simulink model "SHM_900HZ_TG190428test"  (Simulink 7.7)
settings: Solver=ode113  SolverMode=SingleTasking  StartTime=0.0  StopTime=3  RelTol=0.5e-4
undefined symbols (not defined in the file): D11, Delta, SHM900
libraries: powerlib x37, powerlib_extras x22, simulink x6, simulink_extras x1
(part 2 of 2)

== system SHM_900HZ_TG190428test/Controller/PLL/P-I ==
  X : Inport
  Data Type Conversion : DataTypeConversion  SampleTime=TA
  Data Type Conversion3 : DataTypeConversion  SampleTime=TA
  INT1 : Subsystem
  K_i : Gain  Gain=10  SampleTime=TA
  K_p : Gain  SampleTime=TA
  Ki2 : Constant  Value=0.2
  Ki4 : Constant  Value=-0.2
  Logical Operator : Logic  Operator=NOR  AllPortsSameDT=off  OutDataTypeStr=boolean  SampleTime=TA
  Relational Operator : RelationalOperator  OutDataTypeStr=boolean  ZeroCross=off  SampleTime=TA
  Relational Operator1 : RelationalOperator  Operator=<=  OutDataTypeStr=boolean  ZeroCross=off  SampleTime=TA
  Sum2 : Sum  SampleTime=TA
  Switch3 : Switch  Threshold=0.5  ZeroCross=off  SampleTime=TA
  Switch4 : Switch  Threshold=0.5  ZeroCross=off  SampleTime=TA
  Unit Delay : UnitDelay  SampleTime=TA
  Y : Outport
  wires:
  K_p/1 -> Sum2/1
  Sum2/1 -> Relational Operator/1, Switch3/3
  K_i/1 -> INT1/1(x)
  INT1/1(y) -> Sum2/2
  Data Type Conversion/1 -> Switch3/2
  Ki2/1 -> Switch3/1, Relational Operator/2
  Relational Operator/1 -> Data Type Conversion/1, Logical Operator/2
  Switch3/1 -> Switch4/3, Relational Operator1/1
  Ki4/1 -> Switch4/1, Relational Operator1/2
  Relational Operator1/1 -> Data Type Conversion3/1, Logical Operator/1
  Data Type Conversion3/1 -> Switch4/2
  Logical Operator/1 -> Unit Delay/1
  Unit Delay/1 -> INT1/2(S)
  X/1 -> K_p/1, K_i/1
  Switch4/1 -> Y/1

== system SHM_900HZ_TG190428test/Controller/Regulator1/1st order delay1 ==
  x : Inport
  Kd_1 : Gain  Gain=TA/0.005  SampleTime=TA
  Kd_2 : Gain  Gain=0.5  SampleTime=TA
  Sum1 : Sum  SampleTime=TA
  Sum4 : Sum  Inputs=+-  SampleTime=TA
  Sum6 : Sum  SampleTime=TA
  Unit Delay1 : UnitDelay  SampleTime=TA
  y : Outport
  wires:
  Sum4/1 -> Kd_1/1
  Kd_1/1 -> Sum6/1
  Sum6/1 -> Unit Delay1/1, Sum1/1
  Unit Delay1/1 -> Sum6/2, Sum4/2, Sum1/2
  x/1 -> Sum4/1
  Sum1/1 -> Kd_2/1
  Kd_2/1 -> y/1

== system SHM_900HZ_TG190428test/Controller/Regulator1/1st order delay2 ==
  x : Inport
  Kd_1 : Gain  Gain=TA/0.05  SampleTime=TA
  Kd_2 : Gain  Gain=0.5  SampleTime=TA
  Sum1 : Sum  SampleTime=TA
  Sum4 : Sum  Inputs=+-  SampleTime=TA
  Sum6 : Sum  SampleTime=TA
  Unit Delay1 : UnitDelay  SampleTime=TA
  y : Outport
  wires:
  Sum4/1 -> Kd_1/1
  Kd_1/1 -> Sum6/1
  Sum6/1 -> Unit Delay1/1, Sum1/1
  Unit Delay1/1 -> Sum6/2, Sum4/2, Sum1/2
  x/1 -> Sum4/1
  Sum1/1 -> Kd_2/1
  Kd_2/1 -> y/1

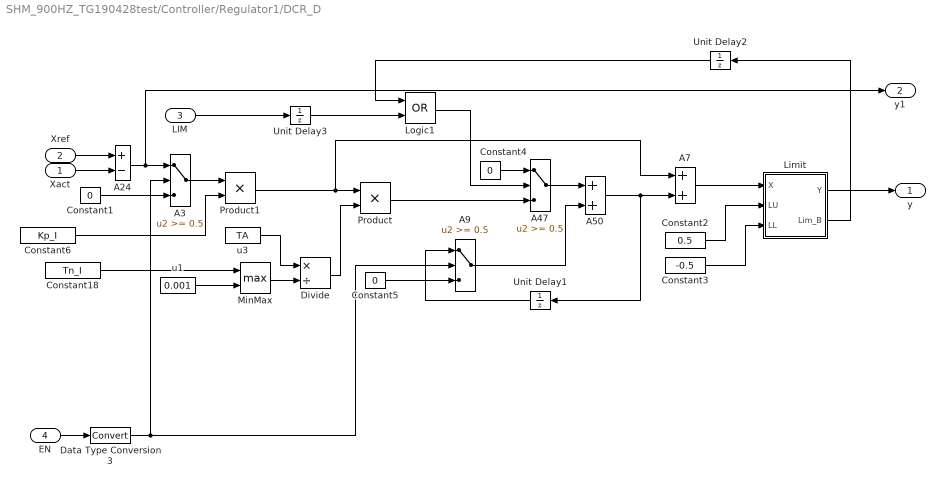
== system SHM_900HZ_TG190428test/Controller/Regulator1/DCR_D ==
  Xact : Inport
  Xref : Inport  Port=2
  LIM : Inport  Port=3
  EN : Inport  Port=4
  A24 : Sum  Inputs=+-  SampleTime=TA
  A3 : Switch  Threshold=0.5  ZeroCross=off
  A47 : Switch  Threshold=0.5  ZeroCross=off
  A50 : Sum  SampleTime=TA
  A7 : Sum  InputSameDT=on
  A9 : Switch  Threshold=0.5  ZeroCross=off
  Constant1 : Constant  Value=0
  Constant18 : Constant  Value=Tn_I
  Constant2 : Constant  Value=0.5
  Constant3 : Constant  Value=-0.5
  Constant4 : Constant  Value=0
  Constant5 : Constant  Value=0
  Constant6 : Constant  Value=Kp_I
  Data Type Conversion3 : DataTypeConversion
  Divide : Product  Inputs=*/
  Limit : Subsystem
  Logic1 : Logic  Operator=OR  AllPortsSameDT=off  OutDataTypeStr=boolean
  MinMax : MinMax  Function=max  Inputs=2
  Product : Product  RndMeth=Zero
  Product1 : Product  RndMeth=Zero
  Unit Delay1 : UnitDelay  SampleTime=-1
  Unit Delay2 : UnitDelay  SampleTime=-1
  Unit Delay3 : UnitDelay  SampleTime=-1
  u1 : Constant  Value=0.001  SampleTime=-1
  u3 : Constant  Value=TA  SampleTime=-1
  y : Outport
  y1 : Outport  Port=2
  wires:
  Divide/1 -> Product/2
  MinMax/1 -> Divide/2
  u1/1 -> MinMax/2
  u3/1 -> Divide/1
  Constant18/1 -> MinMax/1
  Data Type Conversion3/1 -> A3/2, A9/2
  Xact/1 -> A24/2
  Xref/1 -> A24/1
  A24/1 -> A3/1, y1/1
  Constant1/1 -> A3/3
  A3/1 -> Product1/1
  Constant6/1 -> Product1/2
  Product1/1 -> A7/1, Product/1
  Product/1 -> A47/3
  Limit/1(Y) -> y/1
  EN/1 -> Data Type Conversion3/1
  Unit Delay1/1 -> A9/1
  Constant5/1 -> A9/3
  Constant4/1 -> A47/1
  A47/1 -> A50/1
  A9/1 -> A50/2
  A50/1 -> A7/2, Unit Delay1/1
  A7/1 -> Limit/1(X)
  Constant2/1 -> Limit/2(LU)
  Constant3/1 -> Limit/3(LL)
  Limit/2(Lim_B) -> Unit Delay2/1
  Logic1/1 -> A47/2
  Unit Delay2/1 -> Logic1/1
  Unit Delay3/1 -> Logic1/2
  LIM/1 -> Unit Delay3/1

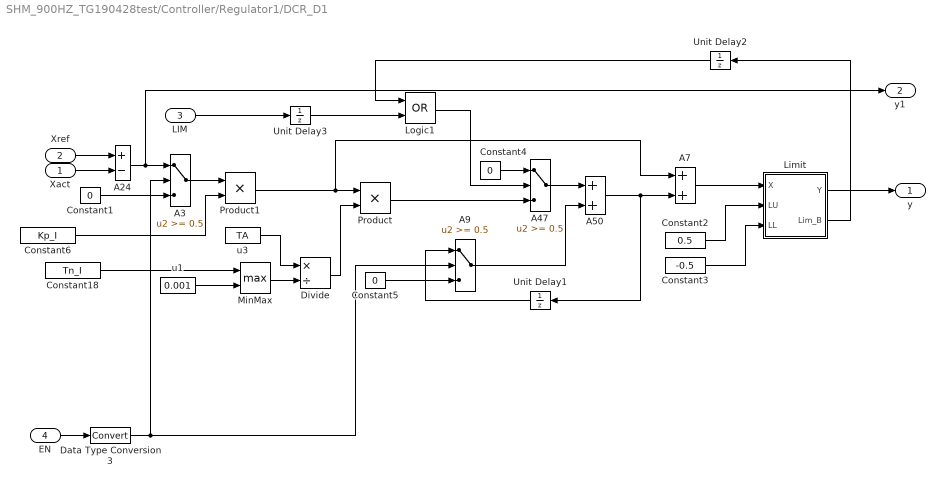
== system SHM_900HZ_TG190428test/Controller/Regulator1/DCR_D1 ==
  Xact : Inport
  Xref : Inport  Port=2
  LIM : Inport  Port=3
  EN : Inport  Port=4
  A24 : Sum  Inputs=+-  SampleTime=TA
  A3 : Switch  Threshold=0.5  ZeroCross=off
  A47 : Switch  Threshold=0.5  ZeroCross=off
  A50 : Sum  SampleTime=TA
  A7 : Sum  InputSameDT=on
  A9 : Switch  Threshold=0.5  ZeroCross=off
  Constant1 : Constant  Value=0
  Constant18 : Constant  Value=Tn_I
  Constant2 : Constant  Value=0.5
  Constant3 : Constant  Value=-0.5
  Constant4 : Constant  Value=0
  Constant5 : Constant  Value=0
  Constant6 : Constant  Value=Kp_I
  Data Type Conversion3 : DataTypeConversion
  Divide : Product  Inputs=*/
  Limit : Subsystem
  Logic1 : Logic  Operator=OR  AllPortsSameDT=off  OutDataTypeStr=boolean
  MinMax : MinMax  Function=max  Inputs=2
  Product : Product  RndMeth=Zero
  Product1 : Product  RndMeth=Zero
  Unit Delay1 : UnitDelay  SampleTime=-1
  Unit Delay2 : UnitDelay  SampleTime=-1
  Unit Delay3 : UnitDelay  SampleTime=-1
  u1 : Constant  Value=0.001  SampleTime=-1
  u3 : Constant  Value=TA  SampleTime=-1
  y : Outport
  y1 : Outport  Port=2
  wires:
  LIM/1 -> Unit Delay3/1
  Unit Delay3/1 -> Logic1/2
  Unit Delay2/1 -> Logic1/1
  Logic1/1 -> A47/2
  Limit/2(Lim_B) -> Unit Delay2/1
  Constant3/1 -> Limit/3(LL)
  Constant2/1 -> Limit/2(LU)
  A7/1 -> Limit/1(X)
  A50/1 -> Unit Delay1/1, A7/2
  A9/1 -> A50/2
  A47/1 -> A50/1
  Constant4/1 -> A47/1
  Constant5/1 -> A9/3
  Unit Delay1/1 -> A9/1
  EN/1 -> Data Type Conversion3/1
  Limit/1(Y) -> y/1
  Product/1 -> A47/3
  Product1/1 -> Product/1, A7/1
  Constant6/1 -> Product1/2
  A3/1 -> Product1/1
  Constant1/1 -> A3/3
  A24/1 -> y1/1, A3/1
  Xref/1 -> A24/1
  Xact/1 -> A24/2
  Data Type Conversion3/1 -> A9/2, A3/2
  Constant18/1 -> MinMax/1
  u3/1 -> Divide/1
  u1/1 -> MinMax/2
  MinMax/1 -> Divide/2
  Divide/1 -> Product/2

== system SHM_900HZ_TG190428test/Controller/Regulator1/DCR_Q ==
  M_max : Inport
  EN : Inport  Port=2
  Constant10 : Constant  Value=0
  Constant11 : Constant  Value=-0.2
  Constant7 : Constant  Value=1.06
  Constant9 : Constant  Value=0.1
  Data Type Conversion3 : DataTypeConversion
  IR : Subsystem
  Iq_resp1 : Scope  NumInputPorts=3
      settings: YMin=-0.375~-0.3~-5  YMax=0.125~0.3~5  SaveName=ScopeData2  SampleInput=on  SampleTime=1E-4
  Unit Delay2 : UnitDelay  SampleTime=-1
  Unit Delay4 : UnitDelay  SampleTime=TA
  Iq_ref : Outport
  wires:
  EN/1 -> Data Type Conversion3/1
  Data Type Conversion3/1 -> IR/6(EN)
  M_max/1 -> IR/2(Xact), Iq_resp1/1
  Constant9/1 -> IR/3(Tn)
  Constant11/1 -> IR/5(LL)
  Constant10/1 -> IR/4(LU)
  Constant7/1 -> IR/1(Xref)
  Unit Delay4/1 -> Iq_resp1/2
  IR/1(yi) -> Unit Delay4/1, Iq_resp1/3, Iq_ref/1

== system SHM_900HZ_TG190428test/Controller/Regulator1/Iq_Dif3 ==
  In1 : Inport
  1st order delay2 : Subsystem
  Iq_resp3 : Scope  NumInputPorts=3
      settings: YMin=-0.375~-0.3~-5  YMax=0.125~0.3~5  SampleInput=on  SampleTime=TA
  Sum1 : Sum  Inputs=+-  SampleTime=TA
  Sum2 : Sum  SampleTime=TA
  Sum3 : Sum  SampleTime=TA
  Unit Delay2 : UnitDelay  SampleTime=TA
  Unit Delay3 : UnitDelay  SampleTime=TA
  V->pu1 : Gain  Gain=Kpre  SampleTime=TA  SaturateOnIntegerOverflow=on  OutDataTypeStr=Inherit: Same as input  ParamDataTypeStr=Inherit: Same as input
  V->pu4 : Gain  Gain=0.5*La/(314*TA)  SampleTime=TA  SaturateOnIntegerOverflow=on  OutDataTypeStr=Inherit: Same as input  ParamDataTypeStr=Inherit: Same as input
  Out1 : Outport
  wires:
  Sum3/1 -> Sum1/2
  Sum2/1 -> Sum1/1
  Unit Delay3/1 -> Sum3/2
  V->pu1/1 -> Iq_resp3/3, Out1/1
  1st order delay2/1(y) -> Iq_resp3/1, Sum2/1, Unit Delay2/1
  Unit Delay2/1 -> Sum3/1, Sum2/2, Unit Delay3/1
  Sum1/1 -> Iq_resp3/2, V->pu4/1
  In1/1 -> 1st order delay2/1(x)
  V->pu4/1 -> V->pu1/1

== system SHM_900HZ_TG190428test/Controller/Regulator1/VD ==
  Fis : Inport
  Iac : Inport  Port=2
  Constant1 : Constant  Value=-TA*fn*2*pi
  Demux2 : Demux  Outputs=3
  Gain2 : Gain  Gain=-1/3  SampleTime=TA
  Gain4 : Gain  Gain=1/sqrt(3)  SampleTime=TA
  Gain5 : Gain  Gain=2/sqrt(3)  SampleTime=TA
  Mux7 : Mux  Inputs=2
  Product{4..7} (4 alike) : Product  SampleTime=TA  RndMeth=Zero
  Sum1 : Sum  Inputs=|++  SampleTime=TA
  Sum2 : Sum  SampleTime=TA
  Sum3 : Sum  Inputs=|+-  SampleTime=TA
  Sum7 : Sum  Inputs=+++  SampleTime=TA
  Sum8 : Sum  Inputs=|++  SampleTime=TA
  Sum9 : Sum  Inputs=+++  SampleTime=TA
  Trigonometric Function1 : Trigonometry  Operator=cos  SampleTime=TA
  Trigonometric Function2 : Trigonometry  SampleTime=TA
  Idq : Outport
  wires:
  Trigonometric Function1/1 -> Product7/2, Product4/2
  Trigonometric Function2/1 -> Product6/2, Product5/2
  Demux2/1 -> Sum8/1, Sum7/1, Gain4/1
  Sum9/1 -> Product7/1, Product5/1
  Product6/1 -> Sum3/1
  Product7/1 -> Sum3/2
  Product4/1 -> Sum1/1
  Product5/1 -> Sum1/2
  Gain4/1 -> Sum9/1
  Gain5/1 -> Sum9/2
  Demux2/2 -> Gain5/1, Sum7/2
  Sum2/1 -> Trigonometric Function2/1, Trigonometric Function1/1
  Sum3/1 -> Mux7/1
  Sum1/1 -> Mux7/2
  Sum8/1 -> Product4/1, Product6/1
  Demux2/3 -> Sum7/3
  Sum7/1 -> Gain2/1
  Gain2/1 -> Sum8/2, Sum9/3
  Constant1/1 -> Sum2/2
  Fis/1 -> Sum2/1
  Iac/1 -> Demux2/1
  Mux7/1 -> Idq/1

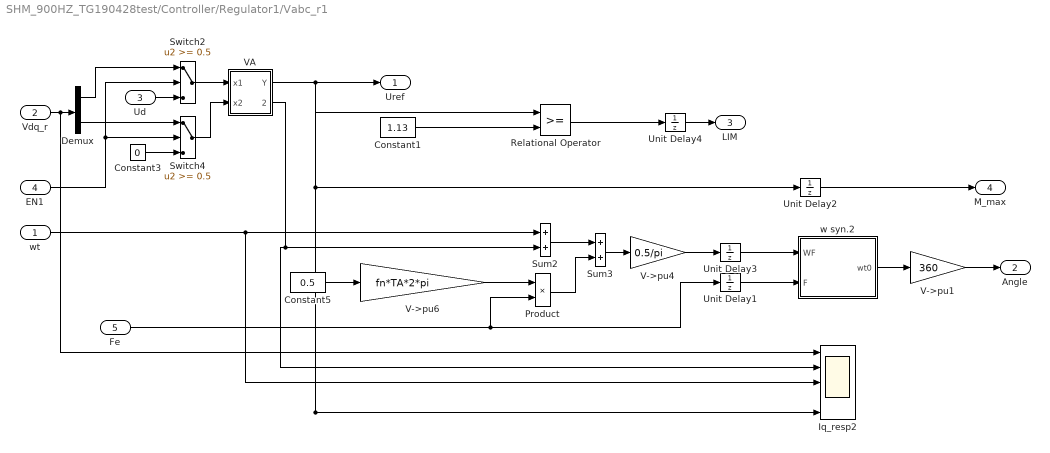
== system SHM_900HZ_TG190428test/Controller/Regulator1/Vabc_r1 ==
  wt : Inport
  Vdq_r : Inport  Port=2
  Ud : Inport  Port=3
  EN1 : Inport  Port=4
  Fe : Inport  Port=5
  Constant1 : Constant  Value=1.13
  Constant3 : Constant  Value=0
  Constant5 : Constant  Value=0.5
  Demux : Demux  Outputs=2
  Iq_resp2 : Scope  NumInputPorts=5
      settings: YMin=-0.375~-0.3~-5~-5~-5  YMax=0.125~0.3~5~5~5  SampleInput=on  SampleTime=1E-4
  Product : Product  SampleTime=TA  RndMeth=Zero
  Relational Operator : RelationalOperator  OutDataTypeStr=boolean
  Sum2 : Sum  SampleTime=TA
  Sum3 : Sum  SampleTime=TA
  Switch2 : Switch  Threshold=0.5  ZeroCross=off  SampleTime=TA
  Switch4 : Switch  Threshold=0.5  ZeroCross=off  SampleTime=TA
  Unit Delay{1..4} (4 alike) : UnitDelay  SampleTime=TA
  V->pu1 : Gain  Gain=360  SampleTime=Ts  SaturateOnIntegerOverflow=on  OutDataTypeStr=Inherit: Same as input  ParamDataTypeStr=Inherit: Same as input
  V->pu4 : Gain  Gain=0.5/pi  SampleTime=TA  SaturateOnIntegerOverflow=on  OutDataTypeStr=Inherit: Same as input  ParamDataTypeStr=Inherit: Same as input
  V->pu6 : Gain  Gain=fn*TA*2*pi  SampleTime=TA  SaturateOnIntegerOverflow=on  OutDataTypeStr=Inherit: Same as input  ParamDataTypeStr=Inherit: Same as input
  VA : Subsystem
  w syn.2 : Subsystem  mask{Ts1=2e-6}
  Uref : Outport
  Angle : Outport  Port=2
  LIM : Outport  Port=3
  M_max : Outport  Port=4
  wires:
  Vdq_r/1 -> Demux/1, Iq_resp2/1
  Sum2/1 -> Sum3/1
  Sum3/1 -> V->pu4/1
  Product/1 -> Sum3/2
  wt/1 -> Sum2/1, Iq_resp2/3
  Switch2/1 -> VA/1(x1)
  Switch4/1 -> VA/2(x2)
  EN1/1 -> Switch4/2, Switch2/2
  Demux/2 -> Switch4/1
  Demux/1 -> Switch2/1
  Ud/1 -> Switch2/3
  Constant3/1 -> Switch4/3
  Constant5/1 -> V->pu6/1
  V->pu6/1 -> Product/1
  Fe/1 -> Product/2, Unit Delay1/1
  VA/2(ang) -> Sum2/2, Iq_resp2/2
  V->pu4/1 -> Unit Delay3/1
  w syn.2/1(wt0) -> V->pu1/1
  V->pu1/1 -> Angle/1
  Unit Delay3/1 -> w syn.2/1(WF)
  Unit Delay1/1 -> w syn.2/2(F)
  VA/1(Y) -> Uref/1, Iq_resp2/5, Relational Operator/1, Unit Delay2/1
  Constant1/1 -> Relational Operator/2
  Relational Operator/1 -> Unit Delay4/1
  Unit Delay2/1 -> M_max/1
  Unit Delay4/1 -> LIM/1

== system SHM_900HZ_TG190428test/Controller/Regulator1/Vdc_reg ==
  Uset : Inport
  Tac : Inport  Port=2
  Idc_L : Inport  Port=3
  Vdc : Inport  Port=4
  LIM : Inport  Port=5
  EN : Inport  Port=6
  Ud_net : Inport  Port=7
  1st order delay1 : Subsystem
  1st order delay2 : Subsystem
  A1 : MinMax  Function=max  Inputs=2  ZeroCross=off  SampleTime=TA
  A3 : MinMax  Inputs=2  ZeroCross=off  SampleTime=TA
  Constant1 : Constant  Value=2.4
  Constant11 : Constant  Value=3.3*1.5/2
  Constant2 : Constant  Value=1.1
  Divide : Product  Inputs=*/
  Product : Product  RndMeth=Zero
  Saturation1 : Saturate  UpperLimit=1.3  LowerLimit=0.9  ZeroCross=off  SampleTime=TA
  Saturation2 : Saturate  UpperLimit=1.3  LowerLimit=0.9  ZeroCross=off  SampleTime=TA
  Uref1 : Subsystem
  controller : Subsystem
  Id_r : Outport
  Vdc1 : Outport  Port=2
  Uref : Outport  Port=3
  wires:
  Saturation1/1 -> Uref1/2(Uact), controller/2(X_act), 1st order delay1/1(x)
  EN/1 -> Uref1/5(EN), controller/4(EN)
  Idc_L/1 -> 1st order delay2/1(x)
  Vdc/1 -> Saturation1/1
  Uset/1 -> A1/2
  Tac/1 -> Uref1/3(Tac)
  1st order delay2/1(y) -> controller/3(PRE)
  controller/1(Iref_set) -> Id_r/1
  1st order delay1/1(y) -> Saturation2/1
  Saturation2/1 -> Vdc1/1
  Ud_net/1 -> Product/2
  Uref1/1(Uref) -> controller/1(X_ref)
  Constant11/1 -> Product/1
  Product/1 -> Divide/1
  Constant1/1 -> Divide/2
  Divide/1 -> A1/1
  A1/1 -> A3/2
  Constant2/1 -> A3/1
  A3/1 -> Uref1/1(Uset), Uref/1
  LIM/1 -> Uref1/4(LIM)

== system SHM_900HZ_TG190428test/Controller/Regulator1/Vdq_r1 ==
  Ud : Inport
  Id_r : Inport  Port=2
  Iq_r : Inport  Port=3
  L_sig : Inport  Port=4
  Vd_d : Inport  Port=5
  Vq_d : Inport  Port=6
  Vdc : Inport  Port=7
  Uset : Inport  Port=8
  Constant5 : Constant  Value=U2
  K1 : Constant  Value=2.98
  Mux : Mux  Inputs=2
  Product{,1,3..5} (5 alike) : Product  SampleTime=TA  RndMeth=Zero
  Product2 : Product  Inputs=*/  SampleTime=TA  RndMeth=Zero
  Sum2 : Sum  Inputs=--  SampleTime=TA
  Sum4 : Sum  Inputs=++-  SampleTime=TA
  Vdq_r : Outport
  Ud1 : Outport  Port=2
  wires:
  L_sig/1 -> Product/2, Product1/1
  Iq_r/1 -> Product/1
  Product1/1 -> Sum2/1
  Vq_d/1 -> Sum2/2
  Product/1 -> Sum4/2
  Vd_d/1 -> Sum4/3
  Ud/1 -> Sum4/1, Product5/1
  Id_r/1 -> Product1/2
  Product4/1 -> Vdq_r/1
  Mux/1 -> Product4/1
  Product3/1 -> Product2/2
  K1/1 -> Product3/1
  Constant5/1 -> Product2/1
  Product2/1 -> Product4/2, Product5/2
  Product5/1 -> Ud1/1
  Sum4/1 -> Mux/1
  Sum2/1 -> Mux/2
  Vdc/1 -> Product3/2

== system SHM_900HZ_TG190428test/Controller/Subsystem/PWM2 ==
  HW : Inport
  Real : Inport  Port=2
  EN : Inport  Port=3
  Constant : Constant  Value=0
  Constant1 : Constant
  Constant2 : Constant  Value=0
  Data Type Conversion{,1..7} (8 alike) : DataTypeConversion  SampleTime=Ts
  Logical Operator2 : Logic  AllPortsSameDT=off  OutDataTypeStr=boolean  SampleTime=Ts
  Logical Operator3 : Logic  Operator=NOT  Inputs=1  AllPortsSameDT=off  OutDataTypeStr=boolean  SampleTime=Ts
  Logical Operator4 : Logic  Operator=NOT  Inputs=1  AllPortsSameDT=off  OutDataTypeStr=boolean  SampleTime=Ts
  Mux1 : Mux
  On/Off Delay{1..2,6..7} (4 alike) : powerlib_extras/Control  Blocks/On//Off Delay  SystemSampleTime=-1  type_delay=On delay  delay=Td  ic=0
  Switch{1..4} (4 alike) : Switch  Threshold=0.5  ZeroCross=off  SampleTime=Ts
  Unit Delay1 : UnitDelay  SampleTime=TA
  P1 : Outport
  wires:
  EN/1 -> Data Type Conversion2/1
  Mux1/1 -> Logical Operator2/1
  Logical Operator2/1 -> Data Type Conversion/1
  Data Type Conversion/1 -> P1/1
  Unit Delay1/1 -> Logical Operator2/2
  Data Type Conversion2/1 -> Unit Delay1/1
  HW/1 -> Switch1/2, Switch3/2, Switch4/2, Switch2/2
  Real/1 -> Data Type Conversion1/1, Data Type Conversion3/1, Switch3/1, Switch2/3  "Ust (3 ph)"
  Constant/1 -> Switch2/1
  Constant1/1 -> Switch1/3, Switch4/1
  Data Type Conversion1/1 -> Logical Operator3/1
  Logical Operator3/1 -> Switch1/1
  Logical Operator4/1 -> Switch4/3
  Data Type Conversion3/1 -> Logical Operator4/1
  Constant2/1 -> Switch3/3
  Switch2/1 -> Data Type Conversion4/1
  Switch1/1 -> Data Type Conversion5/1
  Switch4/1 -> Data Type Conversion6/1
  Switch3/1 -> Data Type Conversion7/1
  On/Off Delay7/1 -> Mux1/4
  On/Off Delay2/1 -> Mux1/3
  On/Off Delay6/1 -> Mux1/2
  On/Off Delay1/1 -> Mux1/1
  Data Type Conversion4/1 -> On/Off Delay1/1
  Data Type Conversion5/1 -> On/Off Delay6/1
  Data Type Conversion6/1 -> On/Off Delay2/1
  Data Type Conversion7/1 -> On/Off Delay7/1

== system SHM_900HZ_TG190428test/Controller/Subsystem1/PWM2 ==
  HW : Inport
  Real : Inport  Port=2
  EN : Inport  Port=3
  Constant : Constant  Value=0
  Constant1 : Constant
  Constant2 : Constant  Value=0
  Data Type Conversion{,1..7} (8 alike) : DataTypeConversion  SampleTime=Ts
  Logical Operator2 : Logic  AllPortsSameDT=off  OutDataTypeStr=boolean  SampleTime=Ts
  Logical Operator3 : Logic  Operator=NOT  Inputs=1  AllPortsSameDT=off  OutDataTypeStr=boolean  SampleTime=Ts
  Logical Operator4 : Logic  Operator=NOT  Inputs=1  AllPortsSameDT=off  OutDataTypeStr=boolean  SampleTime=Ts
  Mux1 : Mux
  On/Off Delay{1..2,6..7} (4 alike) : powerlib_extras/Control  Blocks/On//Off Delay  SystemSampleTime=-1  type_delay=On delay  delay=Td  ic=0
  Switch{1..4} (4 alike) : Switch  Threshold=0.5  ZeroCross=off  SampleTime=Ts
  Unit Delay1 : UnitDelay  SampleTime=TA
  P1 : Outport
  wires:
  Data Type Conversion7/1 -> On/Off Delay7/1
  Data Type Conversion6/1 -> On/Off Delay2/1
  Data Type Conversion5/1 -> On/Off Delay6/1
  Data Type Conversion4/1 -> On/Off Delay1/1
  On/Off Delay1/1 -> Mux1/1
  On/Off Delay6/1 -> Mux1/2
  On/Off Delay2/1 -> Mux1/3
  On/Off Delay7/1 -> Mux1/4
  Switch3/1 -> Data Type Conversion7/1
  Switch4/1 -> Data Type Conversion6/1
  Switch1/1 -> Data Type Conversion5/1
  Switch2/1 -> Data Type Conversion4/1
  Constant2/1 -> Switch3/3
  Data Type Conversion3/1 -> Logical Operator4/1
  Logical Operator4/1 -> Switch4/3
  Logical Operator3/1 -> Switch1/1
  Data Type Conversion1/1 -> Logical Operator3/1
  Constant1/1 -> Switch4/1, Switch1/3
  Constant/1 -> Switch2/1
  Real/1 -> Switch2/3, Switch3/1, Data Type Conversion3/1, Data Type Conversion1/1  "Ust (3 ph)"
  HW/1 -> Switch2/2, Switch4/2, Switch3/2, Switch1/2
  Data Type Conversion2/1 -> Unit Delay1/1
  Unit Delay1/1 -> Logical Operator2/2
  Data Type Conversion/1 -> P1/1
  Logical Operator2/1 -> Data Type Conversion/1
  Mux1/1 -> Logical Operator2/1
  EN/1 -> Data Type Conversion2/1

== system SHM_900HZ_TG190428test/Controller/Subsystem2/PWM2 ==
  HW : Inport
  Real : Inport  Port=2
  EN : Inport  Port=3
  Constant : Constant  Value=0
  Constant1 : Constant
  Constant2 : Constant  Value=0
  Data Type Conversion{,1..7} (8 alike) : DataTypeConversion  SampleTime=Ts
  Logical Operator2 : Logic  AllPortsSameDT=off  OutDataTypeStr=boolean  SampleTime=Ts
  Logical Operator3 : Logic  Operator=NOT  Inputs=1  AllPortsSameDT=off  OutDataTypeStr=boolean  SampleTime=Ts
  Logical Operator4 : Logic  Operator=NOT  Inputs=1  AllPortsSameDT=off  OutDataTypeStr=boolean  SampleTime=Ts
  Mux1 : Mux
  On/Off Delay{1..2,6..7} (4 alike) : powerlib_extras/Control  Blocks/On//Off Delay  SystemSampleTime=-1  type_delay=On delay  delay=Td  ic=0
  Switch{1..4} (4 alike) : Switch  Threshold=0.5  ZeroCross=off  SampleTime=Ts
  Unit Delay1 : UnitDelay  SampleTime=TA
  P1 : Outport
  wires:
  EN/1 -> Data Type Conversion2/1
  Mux1/1 -> Logical Operator2/1
  Logical Operator2/1 -> Data Type Conversion/1
  Data Type Conversion/1 -> P1/1
  Unit Delay1/1 -> Logical Operator2/2
  Data Type Conversion2/1 -> Unit Delay1/1
  HW/1 -> Switch1/2, Switch3/2, Switch4/2, Switch2/2
  Real/1 -> Data Type Conversion1/1, Data Type Conversion3/1, Switch3/1, Switch2/3  "Ust (3 ph)"
  Constant/1 -> Switch2/1
  Constant1/1 -> Switch1/3, Switch4/1
  Data Type Conversion1/1 -> Logical Operator3/1
  Logical Operator3/1 -> Switch1/1
  Logical Operator4/1 -> Switch4/3
  Data Type Conversion3/1 -> Logical Operator4/1
  Constant2/1 -> Switch3/3
  Switch2/1 -> Data Type Conversion4/1
  Switch1/1 -> Data Type Conversion5/1
  Switch4/1 -> Data Type Conversion6/1
  Switch3/1 -> Data Type Conversion7/1
  On/Off Delay7/1 -> Mux1/4
  On/Off Delay2/1 -> Mux1/3
  On/Off Delay6/1 -> Mux1/2
  On/Off Delay1/1 -> Mux1/1
  Data Type Conversion4/1 -> On/Off Delay1/1
  Data Type Conversion5/1 -> On/Off Delay6/1
  Data Type Conversion6/1 -> On/Off Delay2/1
  Data Type Conversion7/1 -> On/Off Delay7/1

== system SHM_900HZ_TG190428test/Controller/PLL/P-I/INT1 ==
  x : Inport
  S : Inport  Port=2  SampleTime=1.6e-3
  Add : Sum  SampleTime=TA
  Data Type Conversion : DataTypeConversion  SampleTime=TA
  Data Type Conversion1 : DataTypeConversion  SampleTime=TA
  Data Type Conversion3 : DataTypeConversion  SampleTime=TA
  Ki1 : Constant  Value=0
  Ki2 : Constant  Value=0.1
  Ki4 : Constant  Value=-0.1
  Relational Operator : RelationalOperator  OutDataTypeStr=boolean  ZeroCross=off  SampleTime=TA
  Relational Operator1 : RelationalOperator  Operator=<=  OutDataTypeStr=boolean  ZeroCross=off  SampleTime=TA
  Switch2 : Switch  Threshold=0.5  ZeroCross=off  SampleTime=TA
  Switch3 : Switch  Threshold=0.5  ZeroCross=off  SampleTime=TA
  Switch4 : Switch  Threshold=0.5  ZeroCross=off  SampleTime=TA
  Unit Delay : UnitDelay  SampleTime=TA
  k : Gain  Gain=TA  SampleTime=TA
  y : Outport
  wires:
  Data Type Conversion1/1 -> Switch2/2
  Data Type Conversion/1 -> Switch3/2
  Ki2/1 -> Switch3/1, Relational Operator/2
  Relational Operator/1 -> Data Type Conversion/1
  Ki1/1 -> Switch2/3
  Unit Delay/1 -> Add/2
  Switch2/1 -> Add/1
  Add/1 -> Switch3/3, Relational Operator/1, Unit Delay/1
  x/1 -> k/1
  Switch3/1 -> Switch4/3, Relational Operator1/1
  Ki4/1 -> Switch4/1, Relational Operator1/2
  Relational Operator1/1 -> Data Type Conversion3/1
  Switch4/1 -> y/1
  Data Type Conversion3/1 -> Switch4/2
  S/1 -> Data Type Conversion1/1
  k/1 -> Switch2/1

== system SHM_900HZ_TG190428test/Controller/Regulator1/DCR_D/Limit ==
  X : Inport
  LU : Inport  Port=2
  LL : Inport  Port=3
  Data Type Conversion1 : DataTypeConversion
  Data Type Conversion2 : DataTypeConversion
  Logic1 : Logic  Operator=OR  AllPortsSameDT=off  OutDataTypeStr=boolean
  Relational Operator1 : RelationalOperator  Operator=>  OutDataTypeStr=boolean  ZeroCross=off  InputSameDT=on
  Relational Operator2 : RelationalOperator  Operator=<  OutDataTypeStr=boolean  ZeroCross=off  InputSameDT=on
  Switch1 : Switch  Criteria=u2 > Threshold  Threshold=0.5  ZeroCross=off
  Switch2 : Switch  Criteria=u2 > Threshold  Threshold=0.5  ZeroCross=off
  Y : Outport
  Lim_B : Outport  Port=2
  wires:
  Data Type Conversion1/1 -> Switch2/2
  Data Type Conversion2/1 -> Switch1/2
  Switch1/1 -> Switch2/3
  Switch2/1 -> Y/1
  Relational Operator2/1 -> Data Type Conversion1/1, Logic1/2
  Relational Operator1/1 -> Data Type Conversion2/1, Logic1/1
  X/1 -> Switch1/3, Relational Operator2/1, Relational Operator1/1
  LU/1 -> Switch1/1, Relational Operator1/2
  LL/1 -> Switch2/1, Relational Operator2/2
  Logic1/1 -> Lim_B/1

== system SHM_900HZ_TG190428test/Controller/Regulator1/DCR_D1/Limit ==
  X : Inport
  LU : Inport  Port=2
  LL : Inport  Port=3
  Data Type Conversion1 : DataTypeConversion
  Data Type Conversion2 : DataTypeConversion
  Logic1 : Logic  Operator=OR  AllPortsSameDT=off  OutDataTypeStr=boolean
  Relational Operator1 : RelationalOperator  Operator=>  OutDataTypeStr=boolean  ZeroCross=off  InputSameDT=on
  Relational Operator2 : RelationalOperator  Operator=<  OutDataTypeStr=boolean  ZeroCross=off  InputSameDT=on
  Switch1 : Switch  Criteria=u2 > Threshold  Threshold=0.5  ZeroCross=off
  Switch2 : Switch  Criteria=u2 > Threshold  Threshold=0.5  ZeroCross=off
  Y : Outport
  Lim_B : Outport  Port=2
  wires:
  Logic1/1 -> Lim_B/1
  LL/1 -> Relational Operator2/2, Switch2/1
  LU/1 -> Relational Operator1/2, Switch1/1
  X/1 -> Relational Operator1/1, Relational Operator2/1, Switch1/3
  Relational Operator1/1 -> Logic1/1, Data Type Conversion2/1
  Relational Operator2/1 -> Logic1/2, Data Type Conversion1/1
  Switch2/1 -> Y/1
  Switch1/1 -> Switch2/3
  Data Type Conversion2/1 -> Switch1/2
  Data Type Conversion1/1 -> Switch2/2

== system SHM_900HZ_TG190428test/Controller/Regulator1/DCR_Q/IR ==
  Xref : Inport
  Xact : Inport  Port=2
  Tn : Inport  Port=3
  LU : Inport  Port=4
  LL : Inport  Port=5
  EN : Inport  Port=6
  A24 : Sum  Inputs=+-  SampleTime=TA
  A3 : Switch  Threshold=0.5  ZeroCross=off
  A50 : Sum  SampleTime=TA
  A9 : Switch  Threshold=0.5  ZeroCross=off
  Constant1 : Constant  Value=0
  Constant5 : Constant  Value=0
  Data Type Conversion3 : DataTypeConversion
  Divide : Product  Inputs=*/
  Iq_resp1 : Scope  NumInputPorts=2
      settings: YMin=-0.375~-0.3  YMax=0.125~0.3  SaveName=ScopeData4  SampleInput=on  SampleTime=1E-4
  MinMax : MinMax  Function=max  Inputs=2
  MinMax1 : MinMax  Function=max  Inputs=2
  MinMax2 : MinMax  Inputs=2
  Product : Product  RndMeth=Zero
  Unit Delay1 : UnitDelay  SampleTime=-1
  u1 : Constant  Value=0.001  SampleTime=-1
  u3 : Constant  Value=TA  SampleTime=-1
  yi : Outport
  wires:
  Divide/1 -> Product/2
  MinMax/1 -> Divide/2
  u1/1 -> MinMax/2
  u3/1 -> Divide/1
  Tn/1 -> MinMax/1
  Data Type Conversion3/1 -> A3/2, A9/2, Iq_resp1/2
  Xact/1 -> A24/2
  Xref/1 -> A24/1
  A24/1 -> A3/1
  Constant1/1 -> A3/3
  A3/1 -> Product/1
  Product/1 -> A50/1
  EN/1 -> Data Type Conversion3/1
  Unit Delay1/1 -> A9/1
  Constant5/1 -> A9/3
  A9/1 -> A50/2
  A50/1 -> MinMax1/1
  LL/1 -> MinMax1/2
  MinMax1/1 -> MinMax2/1
  LU/1 -> MinMax2/2
  MinMax2/1 -> Unit Delay1/1, yi/1, Iq_resp1/1

== system SHM_900HZ_TG190428test/Controller/Regulator1/Iq_Dif3/1st order delay2 ==
  x : Inport
  Kd_1 : Gain  Gain=TA/0.01  SampleTime=TA
  Kd_2 : Gain  Gain=0.5  SampleTime=TA
  Sum1 : Sum  SampleTime=TA
  Sum4 : Sum  Inputs=+-  SampleTime=TA
  Sum6 : Sum  SampleTime=TA
  Unit Delay1 : UnitDelay  SampleTime=TA
  y : Outport
  wires:
  Sum4/1 -> Kd_1/1
  Kd_1/1 -> Sum6/1
  Sum6/1 -> Unit Delay1/1, Sum1/1
  Unit Delay1/1 -> Sum6/2, Sum4/2, Sum1/2
  x/1 -> Sum4/1
  Sum1/1 -> Kd_2/1
  Kd_2/1 -> y/1

== system SHM_900HZ_TG190428test/Controller/Regulator1/Vabc_r1/VA ==
  x1 : Inport
  x2 : Inport  Port=2
  Compare To Constant3 : simulink/Logic and Bit Operations/Compare To Constant  SystemSampleTime=-1  relop=<  const=0  LogicOutDataTypeMode=uint8
  Compare To Constant4 : simulink/Logic and Bit Operations/Compare To Constant  SystemSampleTime=-1  relop=~=  const=0  LogicOutDataTypeMode=uint8
  Constant3 : Constant  Value=1e-5
  Constant4 : Constant  Value=2*pi
  Constant5 : Constant  Value=0
  Data Type Conversion1 : DataTypeConversion  SampleTime=TA
  Data Type Conversion2 : DataTypeConversion  SampleTime=TA
  Logical Operator : Logic  Operator=NOT  Inputs=1  AllPortsSameDT=off  OutDataTypeStr=boolean  SampleTime=TA
  Math Function : Math  Operator=sqrt  SampleTime=TA  SaturateOnIntegerOverflow=on
  MinMax : MinMax  Function=max  Inputs=2  ZeroCross=off  SampleTime=TA
  Product1 : Product  SampleTime=TA  SaturateOnIntegerOverflow=on  InputSameDT=on  OutDataTypeStr=Inherit: Same as first input
  Product3 : Product  SampleTime=TA  SaturateOnIntegerOverflow=on  InputSameDT=on  OutDataTypeStr=Inherit: Same as first input
  Product4 : Product  Inputs=*/  SampleTime=TA  SaturateOnIntegerOverflow=on  InputSameDT=on  OutDataTypeStr=Inherit: Same as first input
  Sum3 : Sum  SampleTime=TA  SaturateOnIntegerOverflow=on  InputSameDT=on  OutDataTypeStr=Inherit: Same as first input
  Sum5 : Sum  Inputs=+-  SampleTime=TA  SaturateOnIntegerOverflow=on  InputSameDT=on  OutDataTypeStr=Inherit: Same as first input
  Switch2 : Switch  Threshold=0.5  ZeroCross=off  SampleTime=TA
  Switch4 : Switch  Threshold=0.5  ZeroCross=off  SampleTime=TA
  Trigonometric Function3 : Trigonometry  Operator=acos  SampleTime=TA
  Y : Outport
  ang : Outport  Port=2
  wires:
  Product1/1 -> Sum3/1
  Product3/1 -> Sum3/2
  Sum3/1 -> Math Function/1
  Math Function/1 -> MinMax/1, Compare To Constant4/1, Y/1
  Constant3/1 -> MinMax/2
  MinMax/1 -> Product4/2
  Product4/1 -> Trigonometric Function3/1
  Compare To Constant3/1 -> Data Type Conversion2/1
  Sum5/1 -> Switch2/1
  Constant4/1 -> Sum5/1
  Compare To Constant4/1 -> Logical Operator/1
  Logical Operator/1 -> Data Type Conversion1/1
  Data Type Conversion1/1 -> Switch4/2
  Constant5/1 -> Switch4/1
  Trigonometric Function3/1 -> Switch4/3
  Switch4/1 -> Switch2/3, Sum5/2
  x1/1 -> Product1/2, Product1/1, Product4/1
  x2/1 -> Product3/1, Product3/2, Compare To Constant3/1
  Switch2/1 -> ang/1
  Data Type Conversion2/1 -> Switch2/2

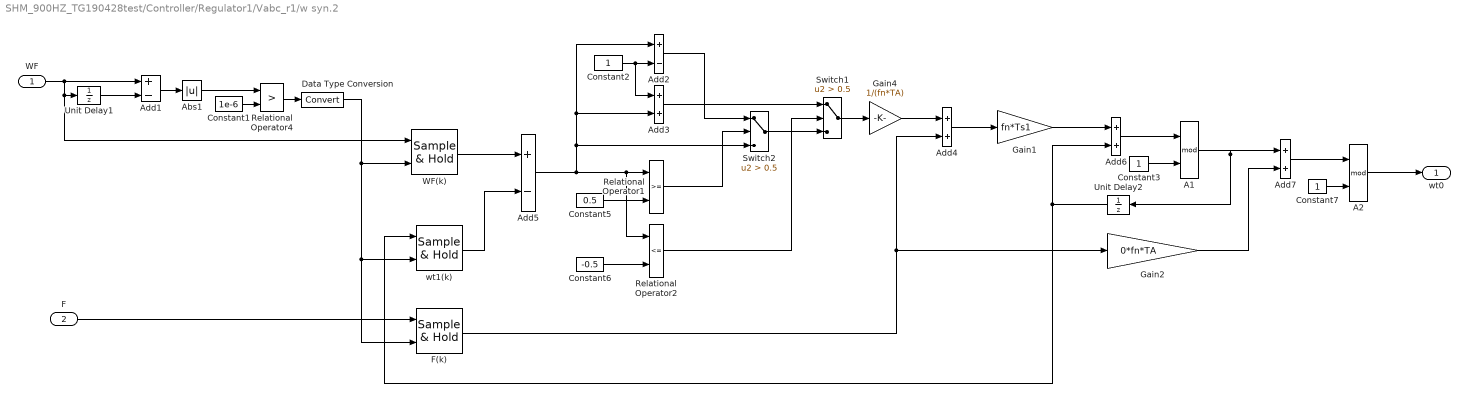
== system SHM_900HZ_TG190428test/Controller/Regulator1/Vabc_r1/w syn.2 ==
  WF : Inport
  F : Inport  Port=2
  A1 : Math  Operator=mod  SampleTime=Ts1  SaturateOnIntegerOverflow=on
  A2 : Math  Operator=mod  SampleTime=Ts1  SaturateOnIntegerOverflow=on
  Abs1 : Abs  ZeroCross=off  SampleTime=Ts1
  Add1 : Sum  Inputs=+-  SampleTime=Ts1
  Add2 : Sum  Inputs=+-  SampleTime=Ts1
  Add{3..4,6..7} (4 alike) : Sum  SampleTime=Ts1
  Add5 : Sum  Inputs=+-  SampleTime=Ts1
  Constant1 : Constant  Value=1e-6
  Constant2 : Constant
  Constant3 : Constant
  Constant5 : Constant  Value=0.5
  Constant6 : Constant  Value=-0.5
  Constant7 : Constant
  Data Type Conversion : DataTypeConversion  SampleTime=Ts1
  F(k) : powerlib_extras/Control  Blocks/Sample & Hold  SystemSampleTime=-1  ic=0
  Gain1 : Gain  Gain=fn*Ts1  SampleTime=Ts1
  Gain2 : Gain  Gain=0*fn*TA  SampleTime=Ts1
  Gain4 : Gain  Gain=1/(fn*TA)  SampleTime=Ts1
  Relational Operator1 : RelationalOperator  OutDataTypeStr=boolean  ZeroCross=off  SampleTime=Ts1  InputSameDT=on
  Relational Operator2 : RelationalOperator  Operator=<=  OutDataTypeStr=boolean  ZeroCross=off  SampleTime=Ts1  InputSameDT=on
  Relational Operator4 : RelationalOperator  Operator=>  OutDataTypeStr=boolean  ZeroCross=off  SampleTime=Ts1  InputSameDT=on
  Switch1 : Switch  Criteria=u2 > Threshold  Threshold=0.5  ZeroCross=off  SampleTime=Ts1
  Switch2 : Switch  Criteria=u2 > Threshold  Threshold=0.5  ZeroCross=off  SampleTime=Ts1
  Unit Delay1 : UnitDelay  SampleTime=Ts1
  Unit Delay2 : UnitDelay  SampleTime=Ts1
  WF(k) : powerlib_extras/Control  Blocks/Sample & Hold  SystemSampleTime=-1  ic=0
  wt1(k) : powerlib_extras/Control  Blocks/Sample & Hold  SystemSampleTime=-1  ic=0
  wt0 : Outport
  wires:
  Relational Operator2/1 -> Switch1/2
  Constant6/1 -> Relational Operator2/2
  Constant5/1 -> Relational Operator1/2
  Add5/1 -> Relational Operator2/1, Relational Operator1/1, Add2/1, Add3/2, Switch2/3
  Data Type Conversion/1 -> WF(k)/2, wt1(k)/2, F(k)/2
  F/1 -> F(k)/1
  Abs1/1 -> Relational Operator4/1
  Relational Operator4/1 -> Data Type Conversion/1
  Constant1/1 -> Relational Operator4/2
  Unit Delay1/1 -> Add1/2
  Add1/1 -> Abs1/1
  WF/1 -> WF(k)/1, Unit Delay1/1, Add1/1
  WF(k)/1 -> Add5/1
  wt1(k)/1 -> Add5/2
  Add2/1 -> Switch2/1
  Relational Operator1/1 -> Switch2/2
  Switch2/1 -> Switch1/3
  Add3/1 -> Switch1/1
  Constant2/1 -> Add2/2, Add3/1
  Switch1/1 -> Gain4/1
  Gain4/1 -> Add4/1
  F(k)/1 -> Add4/2, Gain2/1
  Add4/1 -> Gain1/1
  Gain1/1 -> Add6/1
  Add6/1 -> A1/1
  Constant3/1 -> A1/2
  Unit Delay2/1 -> Add6/2, wt1(k)/1
  A1/1 -> Add7/1, Unit Delay2/1
  Add7/1 -> A2/1
  Gain2/1 -> Add7/2
  A2/1 -> wt0/1
  Constant7/1 -> A2/2

== system SHM_900HZ_TG190428test/Controller/Regulator1/Vdc_reg/1st order delay1 ==
  x : Inport
  Kd_1 : Gain  Gain=TA/0.01  SampleTime=TA
  Kd_2 : Gain  Gain=0.5  SampleTime=TA
  Sum1 : Sum  SampleTime=TA
  Sum4 : Sum  Inputs=+-  SampleTime=TA
  Sum6 : Sum  SampleTime=TA
  Unit Delay1 : UnitDelay  SampleTime=TA
  y : Outport
  wires:
  Kd_2/1 -> y/1
  Sum1/1 -> Kd_2/1
  x/1 -> Sum4/1
  Unit Delay1/1 -> Sum1/2, Sum4/2, Sum6/2
  Sum6/1 -> Sum1/1, Unit Delay1/1
  Kd_1/1 -> Sum6/1
  Sum4/1 -> Kd_1/1

== system SHM_900HZ_TG190428test/Controller/Regulator1/Vdc_reg/1st order delay2 ==
  x : Inport
  Kd_1 : Gain  Gain=TA/0.0034  SampleTime=TA
  Kd_2 : Gain  Gain=0.5  SampleTime=TA
  Sum1 : Sum  SampleTime=TA
  Sum4 : Sum  Inputs=+-  SampleTime=TA
  Sum6 : Sum  SampleTime=TA
  Unit Delay1 : UnitDelay  SampleTime=TA
  y : Outport
  wires:
  Sum4/1 -> Kd_1/1
  Kd_1/1 -> Sum6/1
  Sum6/1 -> Unit Delay1/1, Sum1/1
  Unit Delay1/1 -> Sum6/2, Sum4/2, Sum1/2
  x/1 -> Sum4/1
  Sum1/1 -> Kd_2/1
  Kd_2/1 -> y/1

== system SHM_900HZ_TG190428test/Controller/Regulator1/Vdc_reg/Uref1 ==
  Uset : Inport
  Uact : Inport  Port=2
  Tac : Inport  Port=3
  LIM : Inport  Port=4
  EN : Inport  Port=5
  A27a3 : Switch  Criteria=u2 > Threshold  Threshold=0.5  ZeroCross=off  SampleTime=TA
  A27a4 : Switch  Criteria=u2 > Threshold  Threshold=0.5  ZeroCross=off  SampleTime=TA
  A3 : MinMax  Function=max  Inputs=2  ZeroCross=off  SampleTime=TA
  A4 : MinMax  Inputs=2  ZeroCross=off  SampleTime=TA
  Add2 : Sum  Inputs=+-  SampleTime=TA
  Add8 : Sum  SampleTime=TA
  Constant1 : Constant  Value=0
  Constant11 : Constant  Value=TA
  Data Type Conversion1 : DataTypeConversion  SampleTime=TA
  Data Type Conversion5 : DataTypeConversion  SampleTime=TA
  Gain2 : Gain  Gain=-1
  Logical Operator : Logic  Operator=NOT  AllPortsSameDT=off  OutDataTypeStr=boolean
  Logical Operator1 : Logic  AllPortsSameDT=off  OutDataTypeStr=boolean
  Product4 : Product  Inputs=*/  RndMeth=Zero
  Unit Delay1 : UnitDelay  SampleTime=TA
  Uref : Outport
  wires:
  A4/1 -> A3/1
  Product4/1 -> Gain2/1, A4/2
  Constant11/1 -> Product4/1
  A3/1 -> A27a3/1
  Data Type Conversion5/1 -> A27a4/2, A27a3/2
  EN/1 -> Data Type Conversion1/1
  A27a3/1 -> Add8/1
  Add8/1 -> Unit Delay1/1, Uref/1
  A27a4/1 -> Add8/2
  Unit Delay1/1 -> A27a4/1, Add2/2
  Uset/1 -> Add2/1
  Add2/1 -> A4/1
  Tac/1 -> Product4/2
  Gain2/1 -> A3/2
  Constant1/1 -> A27a4/3
  Uact/1 -> A27a3/3
  LIM/1 -> Logical Operator/1
  Data Type Conversion1/1 -> Logical Operator1/1, Logical Operator1/2
  Logical Operator1/1 -> Data Type Conversion5/1

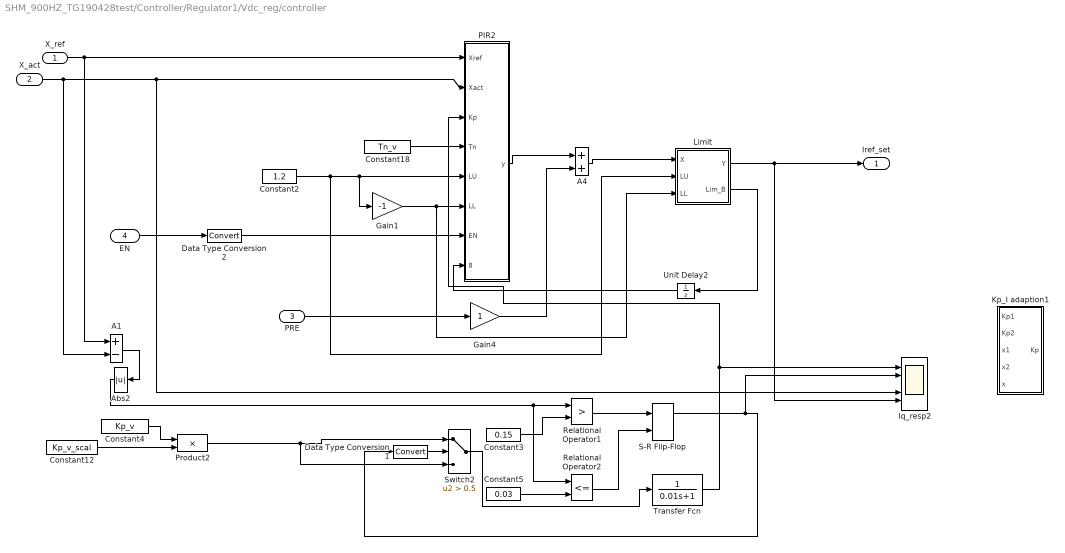
== system SHM_900HZ_TG190428test/Controller/Regulator1/Vdc_reg/controller ==
  X_ref : Inport
  X_act : Inport  Port=2
  PRE : Inport  Port=3
  EN : Inport  Port=4
  A1 : Sum  Inputs=+-  SampleTime=TA
  A4 : Sum  SampleTime=TA
  Abs2 : Abs
  Constant12 : Constant  Value=Kp_v_scal
  Constant18 : Constant  Value=Tn_v
  Constant2 : Constant  Value=1.2
  Constant3 : Constant  Value=0.15
  Constant4 : Constant  Value=Kp_v
  Constant5 : Constant  Value=0.03
  Data Type Conversion1 : DataTypeConversion
  Data Type Conversion2 : DataTypeConversion
  Gain1 : Gain  Gain=-1  SampleTime=TA
  Gain4 : Gain  SampleTime=TA
  Iq_resp2 : Scope  NumInputPorts=5
      settings: YMin=-0.2~-0.25~-0.4~-5~-5  YMax=0.2~0.3~0.5~5~5  SaveName=ScopeData5  SampleInput=on  SampleTime=1E-4
  Kp_I adaption1 : Subsystem
  Limit : Subsystem
  PIR2 : Subsystem
  Product2 : Product  RndMeth=Zero
  Relational Operator1 : RelationalOperator  Operator=>  OutDataTypeStr=boolean  ZeroCross=off  InputSameDT=on
  Relational Operator2 : RelationalOperator  Operator=<=  OutDataTypeStr=boolean  ZeroCross=off  InputSameDT=on
  S-R Flip-Flop : simulink_extras/Flip Flops/S-R Flip-Flop  SystemSampleTime=-1  initial_condition=0
  Switch2 : Switch  Criteria=u2 > Threshold  Threshold=0.5  ZeroCross=off
  Transfer Fcn : TransferFcn  Denominator=[0.01 1]
  Unit Delay2 : UnitDelay  SampleTime=-1
  Iref_set : Outport
  wires:
  EN/1 -> Data Type Conversion2/1
  X_ref/1 -> PIR2/1(Xref), A1/1
  Gain4/1 -> A4/2
  PRE/1 -> Gain4/1
  A4/1 -> Limit/1(X)
  Constant2/1 -> Limit/2(LU), Gain1/1, PIR2/5(LU)
  Data Type Conversion2/1 -> PIR2/7(EN)
  PIR2/1(y) -> A4/1
  X_act/1 -> PIR2/2(Xact), Iq_resp2/4, A1/2
  Limit/1(Y) -> Iref_set/1, Iq_resp2/5
  Limit/2(Lim_B) -> Unit Delay2/1
  Constant18/1 -> PIR2/4(Tn)
  Gain1/1 -> PIR2/6(LL), Limit/3(LL)
  Unit Delay2/1 -> PIR2/8(EN_LIM)
  Constant4/1 -> Product2/1
  Constant12/1 -> Product2/2
  Data Type Conversion1/1 -> Switch2/2
  A1/1 -> Abs2/1
  Constant3/1 -> Relational Operator1/2
  Abs2/1 -> Relational Operator1/1, Relational Operator2/1
  Constant5/1 -> Relational Operator2/2
  Relational Operator1/1 -> S-R Flip-Flop/1
  Relational Operator2/1 -> S-R Flip-Flop/2
  S-R Flip-Flop/1 -> Data Type Conversion1/1, Iq_resp2/2
  Product2/1 -> Switch2/1, Switch2/3
  Switch2/1 -> Transfer Fcn/1
  Transfer Fcn/1 -> PIR2/3(Kp), Iq_resp2/1

== system SHM_900HZ_TG190428test/Controller/Regulator1/Vdc_reg/controller/Kp_I adaption1 ==
  Kp1 : Inport
  Kp2 : Inport  Port=2
  x1 : Inport  Port=3
  x2 : Inport  Port=4
  x : Inport  Port=5
  A10 : Switch  Threshold=0.5  ZeroCross=off
  A11 : Sum  Inputs=+-
  A12 : Sum
  A4 : Switch  Threshold=0.5  ZeroCross=off
  A5 : Switch  Threshold=0.5  ZeroCross=off
  A6 : Sum  Inputs=+-
  A8 : Sum  Inputs=+-
  Abs : Abs
  Divide1 : Product  Inputs=*/
  Product2 : Product  RndMeth=Zero
  Relational Operator1 : RelationalOperator  Operator=<=  OutDataTypeStr=boolean  ZeroCross=off  InputSameDT=on
  Relational Operator3 : RelationalOperator  OutDataTypeStr=boolean  ZeroCross=off  InputSameDT=on
  Relational Operator4 : RelationalOperator  Operator===  OutDataTypeStr=boolean  ZeroCross=off  InputSameDT=on
  u2 : Constant  SampleTime=-1
  Kp : Outport
  wires:
  Abs/1 -> Relational Operator3/1, A11/1, Relational Operator1/1
  A5/1 -> Kp/1
  Product2/1 -> A12/2
  A12/1 -> A4/3
  A11/1 -> Product2/2
  Divide1/1 -> Product2/1
  A4/1 -> A5/3
  x2/1 -> Relational Operator4/2, A8/2, Relational Operator3/2
  A8/1 -> A10/3
  u2/1 -> A10/1
  Relational Operator4/1 -> A10/2
  A10/1 -> Divide1/2
  A6/1 -> Divide1/1
  Kp2/1 -> A5/1, A6/2
  Relational Operator3/1 -> A5/2
  Kp1/1 -> A12/1, A4/1, A6/1
  Relational Operator1/1 -> A4/2
  x/1 -> Abs/1
  x1/1 -> A11/2, Relational Operator4/1, A8/1, Relational Operator1/2

== system SHM_900HZ_TG190428test/Controller/Regulator1/Vdc_reg/controller/Limit ==
  X : Inport
  LU : Inport  Port=2
  LL : Inport  Port=3
  Data Type Conversion1 : DataTypeConversion
  Data Type Conversion2 : DataTypeConversion
  Logic1 : Logic  Operator=OR  AllPortsSameDT=off  OutDataTypeStr=boolean
  Relational Operator1 : RelationalOperator  Operator=>  OutDataTypeStr=boolean  ZeroCross=off  InputSameDT=on
  Relational Operator2 : RelationalOperator  Operator=<  OutDataTypeStr=boolean  ZeroCross=off  InputSameDT=on
  Switch1 : Switch  Criteria=u2 > Threshold  Threshold=0.5  ZeroCross=off
  Switch2 : Switch  Criteria=u2 > Threshold  Threshold=0.5  ZeroCross=off
  Y : Outport
  Lim_B : Outport  Port=2
  wires:
  Data Type Conversion1/1 -> Switch2/2
  Data Type Conversion2/1 -> Switch1/2
  Switch1/1 -> Switch2/3
  Switch2/1 -> Y/1
  Relational Operator2/1 -> Data Type Conversion1/1, Logic1/2
  Relational Operator1/1 -> Data Type Conversion2/1, Logic1/1
  X/1 -> Switch1/3, Relational Operator2/1, Relational Operator1/1
  LU/1 -> Switch1/1, Relational Operator1/2
  LL/1 -> Switch2/1, Relational Operator2/2
  Logic1/1 -> Lim_B/1

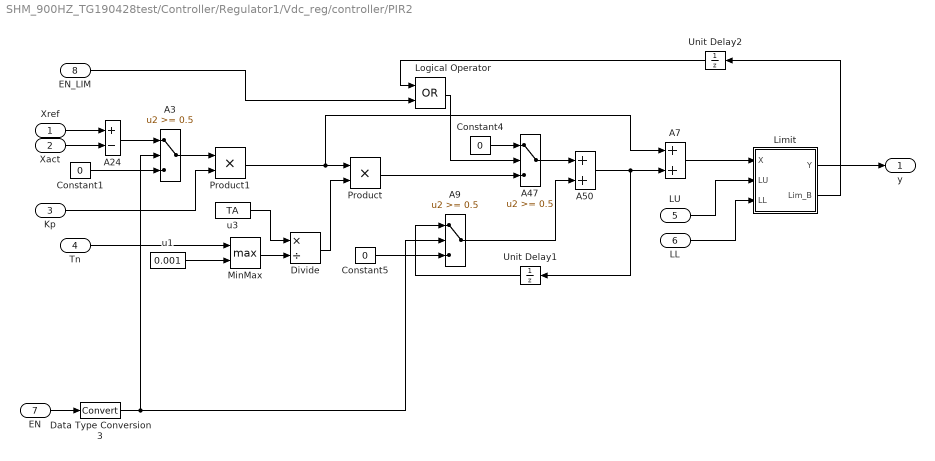
== system SHM_900HZ_TG190428test/Controller/Regulator1/Vdc_reg/controller/PIR2 ==
  Xref : Inport
  Xact : Inport  Port=2
  Kp : Inport  Port=3
  Tn : Inport  Port=4
  LU : Inport  Port=5
  LL : Inport  Port=6
  EN : Inport  Port=7
  EN_LIM : Inport  Port=8
  A24 : Sum  Inputs=+-  SampleTime=TA
  A3 : Switch  Threshold=0.5  ZeroCross=off
  A47 : Switch  Threshold=0.5  ZeroCross=off
  A50 : Sum  SampleTime=TA
  A7 : Sum  InputSameDT=on
  A9 : Switch  Threshold=0.5  ZeroCross=off
  Constant1 : Constant  Value=0
  Constant4 : Constant  Value=0
  Constant5 : Constant  Value=0
  Data Type Conversion3 : DataTypeConversion
  Divide : Product  Inputs=*/
  Limit : Subsystem
  Logical Operator : Logic  Operator=OR  AllPortsSameDT=off  OutDataTypeStr=boolean  SampleTime=TA
  MinMax : MinMax  Function=max  Inputs=2
  Product : Product  RndMeth=Zero
  Product1 : Product  RndMeth=Zero
  Unit Delay1 : UnitDelay  SampleTime=-1
  Unit Delay2 : UnitDelay  SampleTime=-1
  u1 : Constant  Value=0.001  SampleTime=-1
  u3 : Constant  Value=TA  SampleTime=-1
  y : Outport
  wires:
  Divide/1 -> Product/2
  MinMax/1 -> Divide/2
  u1/1 -> MinMax/2
  u3/1 -> Divide/1
  Tn/1 -> MinMax/1
  Data Type Conversion3/1 -> A3/2, A9/2
  Xact/1 -> A24/2
  Xref/1 -> A24/1
  A24/1 -> A3/1
  Constant1/1 -> A3/3
  A3/1 -> Product1/1
  Kp/1 -> Product1/2
  Product1/1 -> Product/1, A7/1
  Product/1 -> A47/3
  Limit/1(Y) -> y/1
  EN/1 -> Data Type Conversion3/1
  Unit Delay1/1 -> A9/1
  Constant5/1 -> A9/3
  Constant4/1 -> A47/1
  A47/1 -> A50/1
  A9/1 -> A50/2
  A50/1 -> A7/2, Unit Delay1/1
  A7/1 -> Limit/1(X)
  LU/1 -> Limit/2(LU)
  LL/1 -> Limit/3(LL)
  Limit/2(Lim_B) -> Unit Delay2/1
  Logical Operator/1 -> A47/2
  Unit Delay2/1 -> Logical Operator/1
  EN_LIM/1 -> Logical Operator/2

== system SHM_900HZ_TG190428test/Controller/Regulator1/Vdc_reg/controller/PIR2/Limit ==
  X : Inport
  LU : Inport  Port=2
  LL : Inport  Port=3
  Data Type Conversion1 : DataTypeConversion
  Data Type Conversion2 : DataTypeConversion
  Logic1 : Logic  Operator=OR  AllPortsSameDT=off  OutDataTypeStr=boolean
  Relational Operator1 : RelationalOperator  Operator=>  OutDataTypeStr=boolean  ZeroCross=off  InputSameDT=on
  Relational Operator2 : RelationalOperator  Operator=<  OutDataTypeStr=boolean  ZeroCross=off  InputSameDT=on
  Switch1 : Switch  Criteria=u2 > Threshold  Threshold=0.5  ZeroCross=off
  Switch2 : Switch  Criteria=u2 > Threshold  Threshold=0.5  ZeroCross=off
  Y : Outport
  Lim_B : Outport  Port=2
  wires:
  Data Type Conversion1/1 -> Switch2/2
  Data Type Conversion2/1 -> Switch1/2
  Switch1/1 -> Switch2/3
  Switch2/1 -> Y/1
  Relational Operator2/1 -> Data Type Conversion1/1, Logic1/2
  Relational Operator1/1 -> Data Type Conversion2/1, Logic1/1
  X/1 -> Switch1/3, Relational Operator2/1, Relational Operator1/1
  LU/1 -> Switch1/1, Relational Operator1/2
  LL/1 -> Switch2/1, Relational Operator2/2
  Logic1/1 -> Lim_B/1
